simulink model "QuadraturePhaseShiftKeying"  (R2018a)
settings: Solver=VariableStepAuto  StartTime=0.0  StopTime=20000  RelTol=1e-3
libraries: commdigbbndpm3 x2, commchan3 x1, commsink2 x1, commrandsrc3 x1
settings Model: Creator=prono  LastModifiedBy=prono

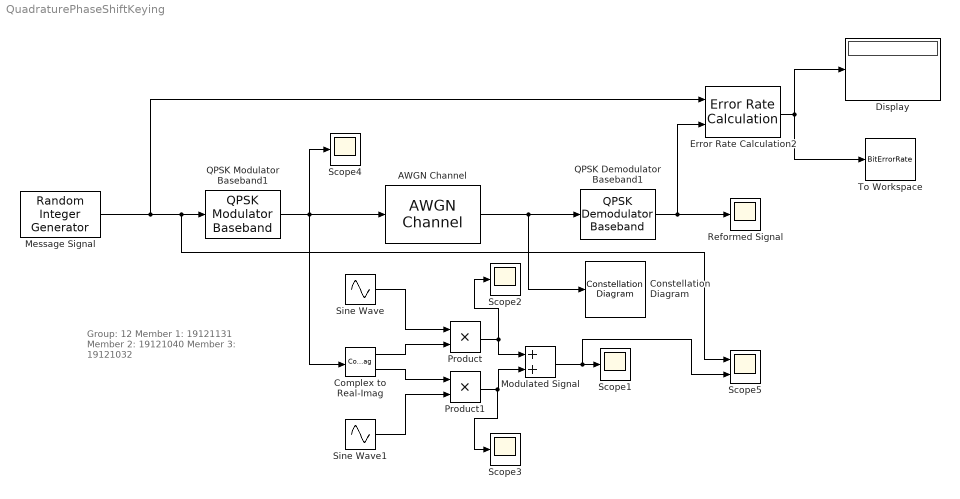
== system QuadraturePhaseShiftKeying ==
  note: Group: 12
      | Member 1: 19121131
      | Member 2: 19121040
      | Member 3: 19121032
  AWGN Channel : commchan3/AWGN Channel  InputProcessing=Columns as channels (frame based)  seed=67  noiseMode="Signal to noise ratio  (Eb/No)"  EbNodB=EbNo  EsNodB=10  SNRdB=10  bitsPerSym=2  Ps=1  Tsym=1  variance=1
  Complex to Real-Imag : ComplexToRealImag
  Constellation Diagram : ConstellationDiagram
  Display : Display
  Error Rate Calculation2 : commsink2/Error Rate Calculation  N=0  st_delay=0  cp_mode=Entire frame  subframe=[]  PMode=Port  WsName=ErrorVec  RsMode2=off  stop=on  numErr=1000  maxBits=1e8
  Message Signal : commrandsrc3/Random Integer Generator  SetSize=4  SeedSource=Auto  Seed=0  SampleTime=0.1  SamplesPerFrame=1  OutputDataType=double  SimulateUsing=Interpreted execution
  Modulated Signal : Sum
  Product : Product
  Product1 : Product
  QPSK Demodulator Baseband1 : commdigbbndpm3/QPSK Demodulator Baseband  OutType=Integer  DecType=Hard decision  VarSource=Dialog  Variance=1  Dec=Gray  Ph=pi/4  outDtype1=Inherit via internal rule  outDtype2=Inherit via internal rule  derotateFactorWordLen=16  derotateFactorDataTypeStr=Inherit: Same word length as input  derotateFactorLastDataTypeStr=Inherit: Same word length as input
  QPSK Modulator Baseband1 : commdigbbndpm3/QPSK Modulator Baseband  InType=Integer  Enc=Gray  Ph=pi/4  outDtype=double  outWordLen=16  outUDDataType=sfix(16)  outFracLenMode=Best precision  outFracLen=15  outDataTypeStr=double  outLastDataTypeStr=double
  Reformed Signal : Scope
  Scope{1..4} (4 alike) : Scope
  Scope5 : Scope  NumInputPorts=2
  Sine Wave : Sin  Frequency=2*pi*5  SampleTime=0.001
  Sine Wave1 : Sin  Frequency=2*pi*5  Phase=pi/2  SampleTime=0.001
  To Workspace : ToWorkspace  VariableName=BitErrorRate  SampleTime=-1
      settings: MaxDataPoints=2  Save2DSignal=2-D array (concatenate along first dimension)
  wires:
  Error Rate Calculation2/1 -> To Workspace/1, Display/1
  AWGN Channel/1 -> QPSK Demodulator Baseband1/1, Constellation Diagram/1
  Modulated Signal/1 -> Scope5/2, Scope1/1
  Product1/1 -> Modulated Signal/2, Scope3/1
  Product/1 -> Modulated Signal/1, Scope2/1
  Sine Wave1/1 -> Product1/2
  Sine Wave/1 -> Product/1
  Complex to Real-Imag/2 -> Product1/1
  Complex to Real-Imag/1 -> Product/2
  QPSK Demodulator Baseband1/1 -> Reformed Signal/1, Error Rate Calculation2/2
  QPSK Modulator Baseband1/1 -> Scope4/1, AWGN Channel/1, Complex to Real-Imag/1
  Message Signal/1 -> Scope5/1, QPSK Modulator Baseband1/1, Error Rate Calculation2/1
